simulink model "Linear_and_Non_linear_model"  (R2024a)
settings: Solver=VariableStepAuto  StartTime=0.0  StopTime=30  RelTol=1e-3
undefined symbols (not defined in the file): D, J_m, K_e, K_t, L_a, N, R_a
libraries: simulink x1
settings Model: PacingRate=0.450000  Creator=tinas  LastModifiedBy=umara

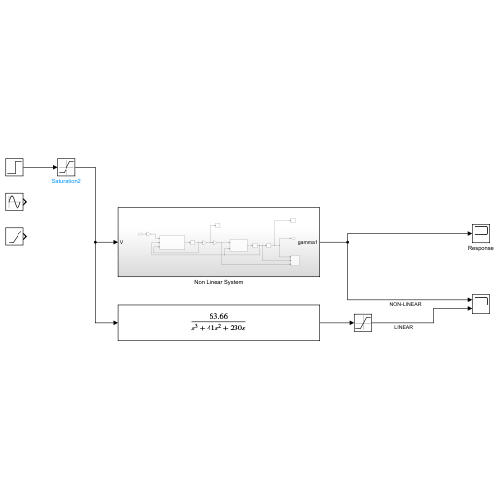
[thumbnail: Simulink's stored preview of the top-level diagram]
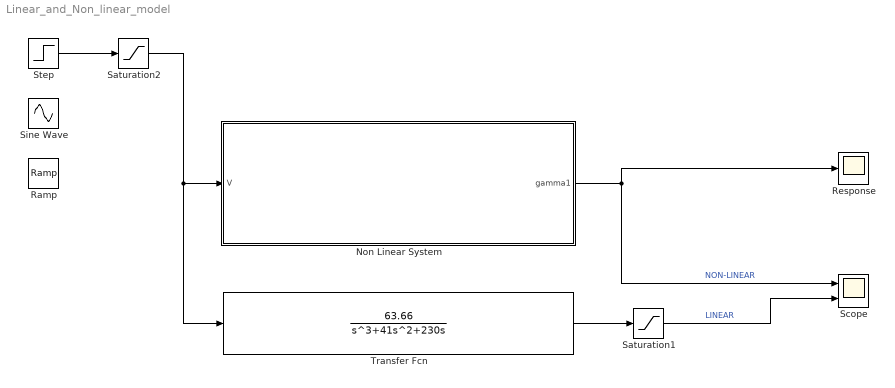
== system Linear_and_Non_linear_model ==
  Non Linear System : Subsystem
  Ramp : simulink/Sources/Ramp  slope=1  start=0  InitialOutput=0
  Response : Scope
  Saturation1 : Saturate  UpperLimit=135*pi/180  LowerLimit=-pi/2
  Saturation2 : Saturate  UpperLimit=12  LowerLimit=-12
  Scope : Scope  NumInputPorts=2
  Sine Wave : Sin  SampleTime=0
  Step : Step  SampleTime=0
  Transfer Fcn : TransferFcn  Numerator=[63.66]  Denominator="[1   41  230  0]"
  wires:
  Step/1 -> Saturation2/1
  Non Linear System/1(gamma1) -> Scope/1, Response/1  "NON-LINEAR"
  Saturation1/1 -> Scope/2  "LINEAR"
  Transfer Fcn/1 -> Saturation1/1
  Saturation2/1 -> Transfer Fcn/1, Non Linear System/1(V)

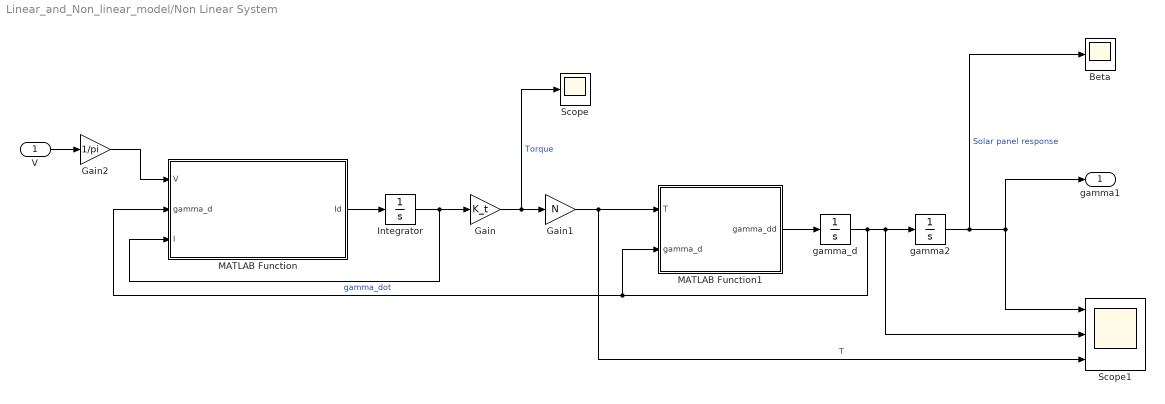
== system Linear_and_Non_linear_model/Non Linear System ==
  V : Inport
  Beta : Scope
  Gain : Gain  Gain=K_t
  Gain1 : Gain  Gain=N
  Gain2 : Gain  Gain=1/pi
  Integrator : Integrator
  MATLAB Function : MATLAB Function  TreatAsAtomicUnit=on
  MATLAB Function1 : MATLAB Function  TreatAsAtomicUnit=on
  Scope : Scope
  Scope1 : Scope  NumInputPorts=3
  gamma2 : Integrator  LimitOutput=on  UpperSaturationLimit=135*pi/180  LowerSaturationLimit=-pi/2
  gamma_d : Integrator
  gamma1 : Outport
  wires:
  Integrator/1 -> Gain/1, MATLAB Function/3(I)
  MATLAB Function1/1(gamma_dd) -> gamma_d/1
  Gain1/1 -> Scope1/3, MATLAB Function1/1(T)  "T"
  gamma2/1 -> Beta/1, gamma1/1, Scope1/1  "Solar panel response"
  gamma_d/1 -> gamma2/1, Scope1/2, MATLAB Function1/2(gamma_d), MATLAB Function/2(gamma_d)  "gamma_dot"
  Gain2/1 -> MATLAB Function/1(V)
  MATLAB Function/1(Id) -> Integrator/1
  Gain/1 -> Gain1/1, Scope/1  "Torque"
  V/1 -> Gain2/1

== matlab function Linear_and_Non_linear_model/Non Linear System/MATLAB Function1 ==
  data: T input; gamma_dd output; gamma_d input; D parameter; J_m parameter
function gamma_dd = fcn(T,gamma_d,D, J_m)

gamma_dd = (T-D*gamma_d)/J_m;


end

== matlab function Linear_and_Non_linear_model/Non Linear System/MATLAB Function ==
  data: V input; Id output; gamma_d input; R_a parameter; K_e parameter; L_a parameter; I input
function Id = fcn(V,gamma_d,R_a, K_e, L_a, I)

 Id=(V-R_a*I- K_e*gamma_d)/L_a;

end
